simulink model "Feedforward_Controller"  (R2024b)
settings: Solver=VariableStepAuto  StartTime=0.0  StopTime=10.0  RelTol=1e-3
values from neighbouring files (symbols this model uses):
  A_rw = [-b/J 0 0 K_t/J 0 0; 0 -b/J 0 0 K_t/J 0; 0 0 -b/J 0 0 K_t/J; -K_e/L 0 0 -R/L 0 0; 0 -K_e/L 0 0 -R/L 0; 0 0 -K_e/L 0 0 -R/L]    [Controller.m]    (also in FeetForward_Controller.mat = [-0.0245517241379 0 0 -20.9439528024 0 0 0 -0.0245517241379 )
  B_rw = [0 0 0; 0 0 0; 0 0 0; 1/L 0 0; 0 1/L 0; 0 0 1/L]    [Controller.m]    (also in FeetForward_Controller.mat = [0 0 0 294.985250737 0 0 0 0 0 0 294.985250737 0 ... (18 ele)
  C_rw = [1 0 0 0 0 0; 0 1 0 0 0 0; 0 0 1 0 0 0]    [Controller.m]    (also in FeetForward_Controller.mat = [1 0 0 0 1 0 0 0 1 0 0 0 ... (18 elements, 3x6)])
  DCM_BODY_wrt_RW = [ 0.408248 0.408248 -0.816496 ... (first row only)    [Controller.m]    (also in FeetForward_Controller.mat = [0.408248  0.408248  -0.816496; -0.7071  0.7071  0; 0.5774  ; ReactionWheelModel1.m)
  I_rw = [I_a 0 0; 0 I_a 0; 0 0 I_a]    [Controller.m]    (also in FeetForward_Controller.mat = [0.0725  0  0; 0  0.0725  0; 0  0  0.0725]; ReactionWheelModel1.m)
  Iab = [Ixx 0 0 ... (first row only)    [Controller.m]    (also in FeetForward_Controller.mat = [4.0774  0  0; 0  4.136  0; 0  0  2.3216]; ReactionWheelModel1.m)
undefined symbols (not defined in the file or in its folder): DiscIntNeverNeededParam
libraries: simulink x18, aerolibutil x1
settings Model: Creator=LEGION  LastModifiedBy=LEGION

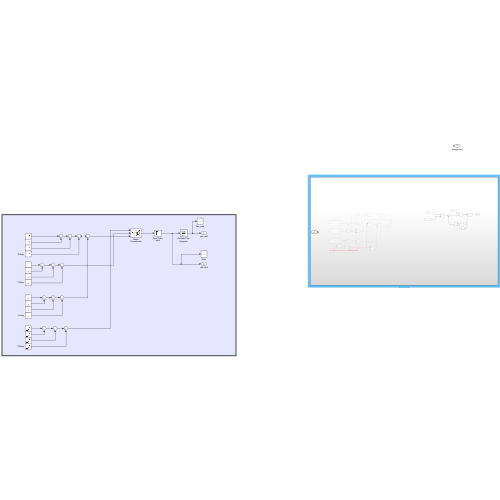
[thumbnail: Simulink's stored preview of the top-level diagram]
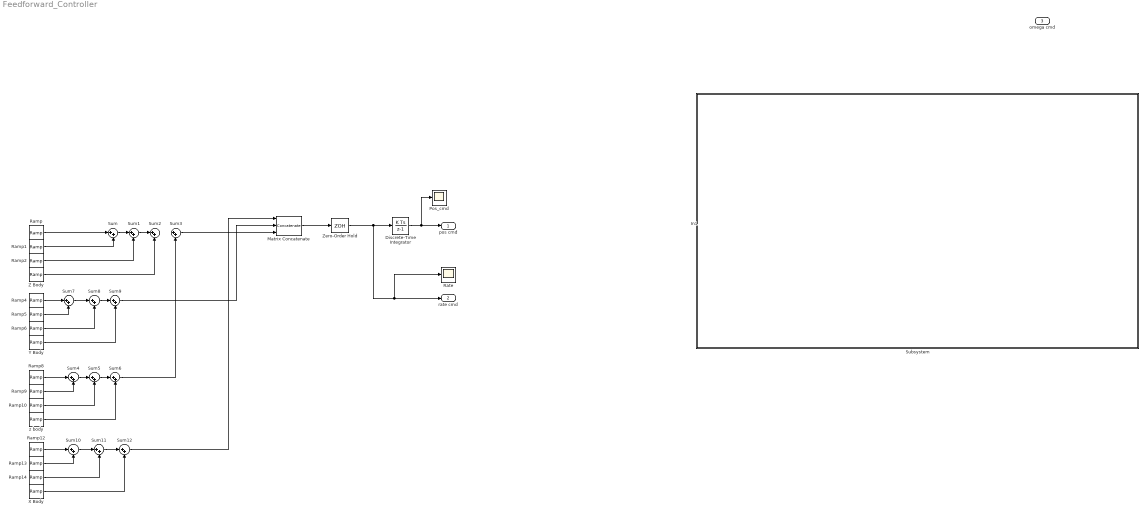
== system Feedforward_Controller ==
  In1 : Inport  Port=2
  Discrete-Time Integrator : DiscreteIntegrator  gainval=1  SampleTime=-1  ICPrevOutput=DiscIntNeverNeededParam  ICPrevScaledInput=DiscIntNeverNeededParam
  Matrix Concatenate : Concatenate  NumInputs=3  Mode=Multidimensional array
  Pos_cmd : Scope
  Ramp{,1..2,4..6,8..10,12..14} (12 alike) : simulink/Sources/Ramp  slope=1  start=0  InitialOutput=0
  Rate : Scope
  Subsystem : Subsystem
  Sum{,1..12} (13 alike) : Sum  Inputs=|++
  X Body : simulink/Sources/Ramp  slope=1  start=0  InitialOutput=0
  Y Body : simulink/Sources/Ramp  slope=1  start=0  InitialOutput=0
  Z Body : simulink/Sources/Ramp  slope=1  start=0  InitialOutput=0
  Zero-Order Hold : ZeroOrderHold
  z body : simulink/Sources/Ramp  slope=1  start=0  InitialOutput=0
  pos cmd : Outport
  rate cmd : Outport  Port=2
  omega cmd : Outport  Port=3
  wires:
  Sum1/1 -> Sum2/1
  Sum/1 -> Sum1/1
  Ramp/1 -> Sum/1
  Ramp1/1 -> Sum/2
  Ramp2/1 -> Sum1/2
  Z Body/1 -> Sum2/2
  Sum5/1 -> Sum6/1
  Sum4/1 -> Sum5/1
  Ramp8/1 -> Sum4/1
  Ramp9/1 -> Sum4/2
  Ramp10/1 -> Sum5/2
  z body/1 -> Sum6/2
  Sum6/1 -> Sum3/2
  Ramp4/1 -> Sum7/1
  Sum7/1 -> Sum8/1
  Sum8/1 -> Sum9/1
  Ramp5/1 -> Sum7/2
  Ramp6/1 -> Sum8/2
  Y Body/1 -> Sum9/2
  Sum3/1 -> Matrix Concatenate/3
  Ramp12/1 -> Sum10/1
  Ramp13/1 -> Sum10/2
  Ramp14/1 -> Sum11/2
  X Body/1 -> Sum12/2
  Sum10/1 -> Sum11/1
  Sum11/1 -> Sum12/1
  Sum12/1 -> Matrix Concatenate/1
  Sum9/1 -> Matrix Concatenate/2
  Matrix Concatenate/1 -> Zero-Order Hold/1
  Zero-Order Hold/1 -> Rate/1, rate cmd/1, Discrete-Time Integrator/1
  Discrete-Time Integrator/1 -> Pos_cmd/1, pos cmd/1

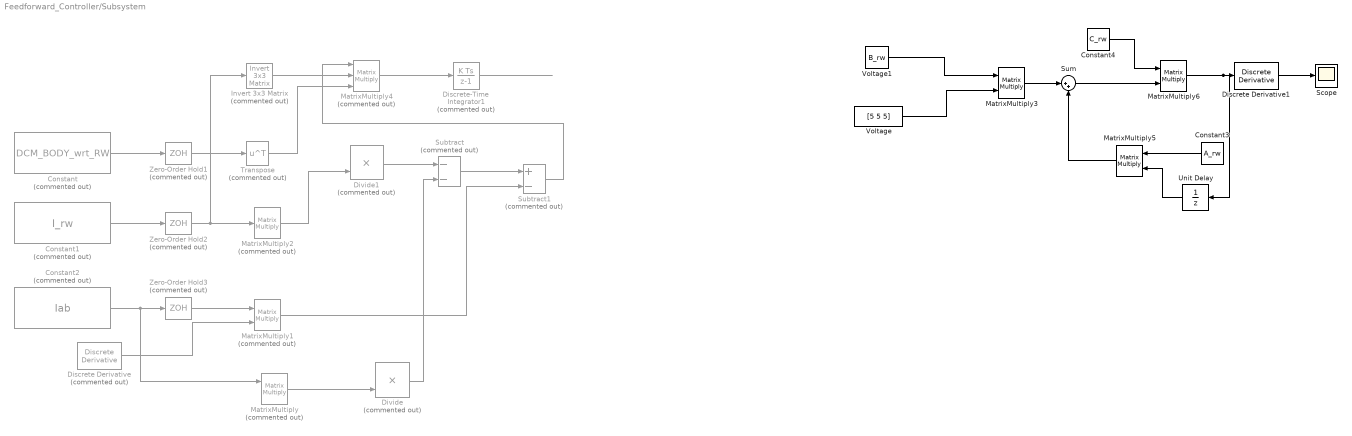
== system Feedforward_Controller/Subsystem ==
  Constant : Constant  Commented=on  Value=DCM_BODY_wrt_RW
  Constant1 : Constant  Commented=on  Value=I_rw
  Constant2 : Constant  Commented=on  Value=Iab
  Constant3 : Constant  Value=A_rw
  Constant4 : Constant  Value=C_rw
  Discrete Derivative : simulink/Discrete/Discrete Derivative  Commented=on  gainval=1.0  ICPrevScaledInput=0.0  OutMin=[]  OutMax=[]  OutDataType=fixdt(1, 16)  OutScaling=2^-10  DoSatur=off
  Discrete Derivative1 : simulink/Discrete/Discrete Derivative  gainval=1.0  ICPrevScaledInput=0.0  OutMin=[]  OutMax=[]  OutDataType=fixdt(1, 16)  OutScaling=2^-10  DoSatur=off
  Discrete-Time Integrator1 : DiscreteIntegrator  Commented=on  SampleTime=-1  ICPrevOutput=DiscIntNeverNeededParam  ICPrevScaledInput=DiscIntNeverNeededParam
  Divide : Product  Commented=on  Inputs=**
  Divide1 : Product  Commented=on  Inputs=**
  Invert 3x3 Matrix : aerolibutil/Invert  3x3 Matrix  Commented=on
  MatrixMultiply : Product  Commented=on  Multiplication=Matrix(*)
  MatrixMultiply1 : Product  Commented=on  Multiplication=Matrix(*)
  MatrixMultiply2 : Product  Commented=on  Inputs=3  Multiplication=Matrix(*)
  MatrixMultiply3 : Product  Multiplication=Matrix(*)
  MatrixMultiply4 : Product  Commented=on  Inputs=3  Multiplication=Matrix(*)
  MatrixMultiply5 : Product  Multiplication=Matrix(*)
  MatrixMultiply6 : Product  Multiplication=Matrix(*)
  Scope : Scope
  Subtract : Sum  Commented=on  Inputs=--
  Subtract1 : Sum  Commented=on  Inputs=+-
  Sum : Sum  Inputs=|++
  Transpose : Math  Commented=on  Operator=transpose
  Unit Delay : UnitDelay  SampleTime=-1  HasFrameUpgradeWarning=on
  Voltage : Constant  Value=[5 5 5]
  Voltage1 : Constant  Value=B_rw
  Zero-Order Hold1 : ZeroOrderHold  Commented=on  SampleTime=-1
  Zero-Order Hold2 : ZeroOrderHold  Commented=on  SampleTime=-1
  Zero-Order Hold3 : ZeroOrderHold  Commented=on  SampleTime=-1
  wires:
  Transpose/1 -> MatrixMultiply4/3
  Zero-Order Hold2/1 -> Invert 3x3 Matrix/1, MatrixMultiply2/2
  Constant2/1 -> Zero-Order Hold3/1, MatrixMultiply/1
  Subtract/1 -> Subtract1/1
  MatrixMultiply4/1 -> Discrete-Time Integrator1/1
  ? -> Divide/1, Divide1/1, MatrixMultiply/2, Discrete Derivative/1
  Discrete-Time Integrator1/1 -> ?
  MatrixMultiply/1 -> Divide/2
  Subtract1/1 -> MatrixMultiply4/1
  Zero-Order Hold3/1 -> MatrixMultiply1/1
  Divide/1 -> Subtract/2
  MatrixMultiply2/1 -> Divide1/2
  Zero-Order Hold1/1 -> Transpose/1
  Constant/1 -> Zero-Order Hold1/1
  Divide1/1 -> Subtract/1
  ? -> MatrixMultiply2/3
  Constant1/1 -> Zero-Order Hold2/1
  MatrixMultiply1/1 -> Subtract1/2
  Discrete Derivative/1 -> MatrixMultiply1/2
  Invert 3x3 Matrix/1 -> MatrixMultiply4/2
  ? -> MatrixMultiply2/1
  Voltage1/1 -> MatrixMultiply3/1
  Voltage/1 -> MatrixMultiply3/2
  MatrixMultiply3/1 -> Sum/1
  MatrixMultiply5/1 -> Sum/2
  Constant3/1 -> MatrixMultiply5/1
  Sum/1 -> MatrixMultiply6/2
  Constant4/1 -> MatrixMultiply6/1
  MatrixMultiply6/1 -> Unit Delay/1, Discrete Derivative1/1
  Discrete Derivative1/1 -> Scope/1
  Unit Delay/1 -> MatrixMultiply5/2
